simulink model "case7"  (R2024b)
settings: Solver=FixedStepAuto  StartTime=0  StopTime=1  FixedStep=1e-7  RelTol=1e-3
values from neighbouring files (symbols this model uses):
  SG_D_1_D = 0.01056    [IEEE9_case_parameters.m]    (also in case1_parameters.m; case2_parameters.m; case3_parameters.m; case4_parameters.m)
  SG_D_1_EnableSaturation = 0    [IEEE9_case_parameters.m]    (also in case1_parameters.m; case2_parameters.m; case3_parameters.m; case4_parameters.m)
  SG_D_1_f0 = 60    [IEEE9_case_parameters.m]    (also in case1_parameters.m; case2_parameters.m; case3_parameters.m; case4_parameters.m)
  SG_D_1_H = 7.5    [IEEE9_case_parameters.m]    (also in case1_parameters.m; case2_parameters.m; case3_parameters.m; case4_parameters.m)
  SG_D_1_K_A = 20    [IEEE9_case_parameters.m]    (also in case1_parameters.m; case2_parameters.m; case3_parameters.m; case4_parameters.m)
  SG_D_1_K_E = 1.000000e+1    (= 10)    [IEEE9_case_parameters.m]    (also in case1_parameters.m; case2_parameters.m; case3_parameters.m; case4_parameters.m)
  SG_D_1_K_F = 2.363    [IEEE9_case_parameters.m]    (also in case1_parameters.m; case2_parameters.m; case3_parameters.m; case4_parameters.m)
  SG_D_1_K_s = 0.5    [IEEE9_case_parameters.m]    (also in case1_parameters.m = 5; case2_parameters.m = 5; case3_parameters.m = 5; case4_parameters.m = 5)
  SG_D_1_R_a = 0.001088    [IEEE9_case_parameters.m]    (also in case1_parameters.m; case2_parameters.m; case3_parameters.m; case4_parameters.m)
  SG_D_1_S_A = 1    [IEEE9_case_parameters.m]    (also in case1_parameters.m; case2_parameters.m; case3_parameters.m; case4_parameters.m)
  SG_D_1_S_B = 0.103    [IEEE9_case_parameters.m]    (also in case1_parameters.m; case2_parameters.m; case3_parameters.m; case4_parameters.m)
  SG_D_1_S_N = 10.659857    [IEEE9_case_parameters.m]    (also in case1_parameters.m; case2_parameters.m; case3_parameters.m; case4_parameters.m)
  SG_D_1_SpeedPara = 200    [IEEE9_case_parameters.m]    (also in case1_parameters.m; case2_parameters.m; case3_parameters.m; case4_parameters.m)
  SG_D_1_T_0 = 0.720173    [IEEE9_case_parameters.m]    (also in case1_parameters.m = 0.755522; case2_parameters.m = 0.808931; case3_parameters.m = 0.869402; case4_parameters.m = 0.729316)
  SG_D_1_T_1 = 0.3    [IEEE9_case_parameters.m]    (also in case1_parameters.m; case2_parameters.m; case3_parameters.m; case4_parameters.m)
  SG_D_1_T_2 = 0.05    [IEEE9_case_parameters.m]    (also in case1_parameters.m; case2_parameters.m; case3_parameters.m; case4_parameters.m)
  SG_D_1_T_3 = 0.02    [IEEE9_case_parameters.m]    (also in case1_parameters.m; case2_parameters.m; case3_parameters.m; case4_parameters.m)
  SG_D_1_T_4 = 0.005    [IEEE9_case_parameters.m]    (also in case1_parameters.m; case2_parameters.m; case3_parameters.m; case4_parameters.m)
  SG_D_1_T_A = 0.02    [IEEE9_case_parameters.m]    (also in case1_parameters.m; case2_parameters.m; case3_parameters.m; case4_parameters.m)
  SG_D_1_T_dd = 8.000000e+0    (= 8)    [IEEE9_case_parameters.m]    (also in case1_parameters.m; case2_parameters.m; case3_parameters.m; case4_parameters.m)
  SG_D_1_T_ddd = 0.04    [IEEE9_case_parameters.m]    (also in case1_parameters.m; case2_parameters.m; case3_parameters.m; case4_parameters.m)
  SG_D_1_T_E = 0.314    [IEEE9_case_parameters.m]    (also in case1_parameters.m; case2_parameters.m; case3_parameters.m; case4_parameters.m)
  SG_D_1_T_F = 0.35    [IEEE9_case_parameters.m]    (also in case1_parameters.m; case2_parameters.m; case3_parameters.m; case4_parameters.m)
  SG_D_1_T_qd = 0.8    [IEEE9_case_parameters.m]    (also in case1_parameters.m; case2_parameters.m; case3_parameters.m; case4_parameters.m)
  SG_D_1_T_qdd = 0.02    [IEEE9_case_parameters.m]    (also in case1_parameters.m; case2_parameters.m; case3_parameters.m; case4_parameters.m)
  SG_D_1_T_speed = 0.1    [IEEE9_case_parameters.m]    (also in case1_parameters.m = 200; case2_parameters.m = 200; case3_parameters.m = 200; case4_parameters.m = 200)
  SG_D_1_T_w = 0.5    [IEEE9_case_parameters.m]    (also in case1_parameters.m; case2_parameters.m; case3_parameters.m; case4_parameters.m)
  SG_D_1_V_ref = 1.990276    [IEEE9_case_parameters.m]    (also in case1_parameters.m = 2.042296; case2_parameters.m = 2.051388; case3_parameters.m = 2.089584; case4_parameters.m = 2.01845)
  SG_D_1_w_ref = 376.991118    [IEEE9_case_parameters.m]    (also in case1_parameters.m; case2_parameters.m; case3_parameters.m; case4_parameters.m)
  SG_D_1_wb = 6.000000e+1    (= 60)    [IEEE9_case_parameters.m]    (also in case1_parameters.m; case2_parameters.m; case3_parameters.m; case4_parameters.m)
  SG_D_1_x_d = 1.9    [IEEE9_case_parameters.m]    (also in case1_parameters.m; case2_parameters.m; case3_parameters.m; case4_parameters.m)
  SG_D_1_x_dd = 0.302    [IEEE9_case_parameters.m]    (also in case1_parameters.m; case2_parameters.m; case3_parameters.m; case4_parameters.m)
  SG_D_1_x_ddd = 0.204    [IEEE9_case_parameters.m]    (also in case1_parameters.m; case2_parameters.m; case3_parameters.m; case4_parameters.m)
  SG_D_1_x_l = 0.05    [IEEE9_case_parameters.m]    (also in case1_parameters.m; case2_parameters.m; case3_parameters.m; case4_parameters.m)
  SG_D_1_x_q = 1.3    [IEEE9_case_parameters.m]    (also in case1_parameters.m; case2_parameters.m; case3_parameters.m; case4_parameters.m)
  SG_D_1_x_qd = 0.5    [IEEE9_case_parameters.m]    (also in case1_parameters.m; case2_parameters.m; case3_parameters.m; case4_parameters.m)
  SG_D_1_x_qdd = 0.3    [IEEE9_case_parameters.m]    (also in case1_parameters.m; case2_parameters.m; case3_parameters.m; case4_parameters.m)
  SG_D_2_D = 0.02    [IEEE9_case_parameters.m]    (also in case1_parameters.m; case2_parameters.m; case3_parameters.m; case4_parameters.m)
  SG_D_2_EnableSaturation = 0    [IEEE9_case_parameters.m]    (also in case1_parameters.m; case2_parameters.m; case3_parameters.m; case4_parameters.m)
  SG_D_2_f0 = 60    [IEEE9_case_parameters.m]    (also in case1_parameters.m; case2_parameters.m; case3_parameters.m; case4_parameters.m)
  SG_D_2_H = 8.000000e+0    (= 8)    [IEEE9_case_parameters.m]    (also in case1_parameters.m; case2_parameters.m; case3_parameters.m; case4_parameters.m)
  SG_D_2_K_A = 20    [IEEE9_case_parameters.m]    (also in case1_parameters.m; case2_parameters.m; case3_parameters.m; case4_parameters.m)
  SG_D_2_K_E = 1.000000e+1    (= 10)    [IEEE9_case_parameters.m]    (also in case1_parameters.m; case2_parameters.m; case3_parameters.m; case4_parameters.m)
  SG_D_2_K_F = 2.363    [IEEE9_case_parameters.m]    (also in case1_parameters.m; case2_parameters.m; case3_parameters.m; case4_parameters.m)
  SG_D_2_K_s = 0.5    [IEEE9_case_parameters.m]    (also in case1_parameters.m = 4; case2_parameters.m = 4; case3_parameters.m = 4; case4_parameters.m = 4)
  SG_D_2_R_a = 0.001088    [IEEE9_case_parameters.m]    (also in case1_parameters.m; case2_parameters.m; case3_parameters.m; case4_parameters.m)
  SG_D_2_S_A = 1    [IEEE9_case_parameters.m]    (also in case1_parameters.m; case2_parameters.m; case3_parameters.m; case4_parameters.m)
  SG_D_2_S_B = 0.103    [IEEE9_case_parameters.m]    (also in case1_parameters.m; case2_parameters.m; case3_parameters.m; case4_parameters.m)
  SG_D_2_S_N = 10.659857    [IEEE9_case_parameters.m]    (also in case1_parameters.m; case2_parameters.m; case3_parameters.m; case4_parameters.m)
  SG_D_2_SpeedPara = 200    [IEEE9_case_parameters.m]    (also in case1_parameters.m; case2_parameters.m; case3_parameters.m; case4_parameters.m)
  SG_D_2_T_0 = 1.632913    [IEEE9_case_parameters.m]    (also in case1_parameters.m = 1.632925; case2_parameters.m = 1.632915; case3_parameters.m = 1.632914; case4_parameters.m = 1.632927)
  SG_D_2_T_1 = 0.2    [IEEE9_case_parameters.m]    (also in case1_parameters.m; case2_parameters.m; case3_parameters.m; case4_parameters.m)
  SG_D_2_T_2 = 0.05    [IEEE9_case_parameters.m]    (also in case1_parameters.m; case2_parameters.m; case3_parameters.m; case4_parameters.m)
  SG_D_2_T_3 = 0.02    [IEEE9_case_parameters.m]    (also in case1_parameters.m; case2_parameters.m; case3_parameters.m; case4_parameters.m)
  SG_D_2_T_4 = 0.005    [IEEE9_case_parameters.m]    (also in case1_parameters.m; case2_parameters.m; case3_parameters.m; case4_parameters.m)
  SG_D_2_T_A = 0.02    [IEEE9_case_parameters.m]    (also in case1_parameters.m; case2_parameters.m; case3_parameters.m; case4_parameters.m)
  SG_D_2_T_dd = 7.9    [IEEE9_case_parameters.m]    (also in case1_parameters.m; case2_parameters.m; case3_parameters.m; case4_parameters.m)
  SG_D_2_T_ddd = 0.04    [IEEE9_case_parameters.m]    (also in case1_parameters.m; case2_parameters.m; case3_parameters.m; case4_parameters.m)
  SG_D_2_T_E = 0.314    [IEEE9_case_parameters.m]    (also in case1_parameters.m; case2_parameters.m; case3_parameters.m; case4_parameters.m)
  SG_D_2_T_F = 0.35    [IEEE9_case_parameters.m]    (also in case1_parameters.m; case2_parameters.m; case3_parameters.m; case4_parameters.m)
  SG_D_2_T_qd = 0.8    [IEEE9_case_parameters.m]    (also in case1_parameters.m; case2_parameters.m; case3_parameters.m; case4_parameters.m)
  SG_D_2_T_qdd = 0.015    [IEEE9_case_parameters.m]    (also in case1_parameters.m; case2_parameters.m; case3_parameters.m; case4_parameters.m)
  SG_D_2_T_speed = 0.1    [IEEE9_case_parameters.m]    (also in case1_parameters.m = 150; case2_parameters.m = 150; case3_parameters.m = 150; case4_parameters.m = 150)
  SG_D_2_T_w = 0.35    [IEEE9_case_parameters.m]    (also in case1_parameters.m; case2_parameters.m; case3_parameters.m; case4_parameters.m)
  SG_D_2_V_ref = 2.58547    [IEEE9_case_parameters.m]    (also in case1_parameters.m = 2.597896; case2_parameters.m = 2.587136; case3_parameters.m = 2.586042; case4_parameters.m = 2.599679)
  SG_D_2_w_ref = 376.991118    [IEEE9_case_parameters.m]    (also in case1_parameters.m; case2_parameters.m; case3_parameters.m; case4_parameters.m)
  SG_D_2_wb = 6.000000e+1    (= 60)    [IEEE9_case_parameters.m]    (also in case1_parameters.m; case2_parameters.m; case3_parameters.m; case4_parameters.m)
  SG_D_2_x_d = 1.8    [IEEE9_case_parameters.m]    (also in case1_parameters.m; case2_parameters.m; case3_parameters.m; case4_parameters.m)
  SG_D_2_x_dd = 0.302    [IEEE9_case_parameters.m]    (also in case1_parameters.m; case2_parameters.m; case3_parameters.m; case4_parameters.m)
  SG_D_2_x_ddd = 0.204    [IEEE9_case_parameters.m]    (also in case1_parameters.m; case2_parameters.m; case3_parameters.m; case4_parameters.m)
  SG_D_2_x_l = 0.05    [IEEE9_case_parameters.m]    (also in case1_parameters.m; case2_parameters.m; case3_parameters.m; case4_parameters.m)
  SG_D_2_x_q = 1.25    [IEEE9_case_parameters.m]    (also in case1_parameters.m; case2_parameters.m; case3_parameters.m; case4_parameters.m)
  SG_D_2_x_qd = 0.5    [IEEE9_case_parameters.m]    (also in case1_parameters.m; case2_parameters.m; case3_parameters.m; case4_parameters.m)
  SG_D_2_x_qdd = 0.3    [IEEE9_case_parameters.m]    (also in case1_parameters.m; case2_parameters.m; case3_parameters.m; case4_parameters.m)
  SG_D_3_D = 0.02    [IEEE9_case_parameters.m]    (also in case1_parameters.m; case2_parameters.m; case3_parameters.m; case4_parameters.m)
  SG_D_3_EnableSaturation = 0    [IEEE9_case_parameters.m]    (also in case1_parameters.m; case2_parameters.m; case3_parameters.m; case4_parameters.m)
  SG_D_3_f0 = 60    [IEEE9_case_parameters.m]    (also in case1_parameters.m; case2_parameters.m; case3_parameters.m; case4_parameters.m)
  SG_D_3_H = 7.7    [IEEE9_case_parameters.m]    (also in case1_parameters.m; case2_parameters.m; case3_parameters.m; case4_parameters.m)
  SG_D_3_K_A = 20    [IEEE9_case_parameters.m]    (also in case1_parameters.m; case2_parameters.m; case3_parameters.m; case4_parameters.m)
  SG_D_3_K_E = 1.000000e+1    (= 10)    [IEEE9_case_parameters.m]    (also in case1_parameters.m; case2_parameters.m; case3_parameters.m; case4_parameters.m)
  SG_D_3_K_F = 2.363    [IEEE9_case_parameters.m]    (also in case1_parameters.m; case2_parameters.m; case3_parameters.m; case4_parameters.m)
  SG_D_3_K_s = 0.2    [IEEE9_case_parameters.m]    (also in case1_parameters.m = 2; case2_parameters.m = 2; case3_parameters.m = 2; case4_parameters.m = 2)
  SG_D_3_R_a = 0.001088    [IEEE9_case_parameters.m]    (also in case1_parameters.m; case2_parameters.m; case3_parameters.m; case4_parameters.m)
  SG_D_3_S_A = 1    [IEEE9_case_parameters.m]    (also in case1_parameters.m; case2_parameters.m; case3_parameters.m; case4_parameters.m)
  SG_D_3_S_B = 0.103    [IEEE9_case_parameters.m]    (also in case1_parameters.m; case2_parameters.m; case3_parameters.m; case4_parameters.m)
  SG_D_3_S_N = 10.659857    [IEEE9_case_parameters.m]    (also in case1_parameters.m; case2_parameters.m; case3_parameters.m; case4_parameters.m)
  SG_D_3_SpeedPara = 200    [IEEE9_case_parameters.m]    (also in case1_parameters.m; case2_parameters.m; case3_parameters.m; case4_parameters.m)
  SG_D_3_T_0 = 0.850788    [IEEE9_case_parameters.m]    (also in case1_parameters.m = 0.850786; case2_parameters.m = 0.850787; case3_parameters.m; case4_parameters.m = 0.850786)
  SG_D_3_T_1 = 0.2    [IEEE9_case_parameters.m]    (also in case1_parameters.m; case2_parameters.m; case3_parameters.m; case4_parameters.m)
  SG_D_3_T_2 = 0.05    [IEEE9_case_parameters.m]    (also in case1_parameters.m; case2_parameters.m; case3_parameters.m; case4_parameters.m)
  SG_D_3_T_3 = 0.02    [IEEE9_case_parameters.m]    (also in case1_parameters.m; case2_parameters.m; case3_parameters.m; case4_parameters.m)
  SG_D_3_T_4 = 0.005    [IEEE9_case_parameters.m]    (also in case1_parameters.m; case2_parameters.m; case3_parameters.m; case4_parameters.m)
  SG_D_3_T_A = 0.02    [IEEE9_case_parameters.m]    (also in case1_parameters.m; case2_parameters.m; case3_parameters.m; case4_parameters.m)
  SG_D_3_T_dd = 8.1    [IEEE9_case_parameters.m]    (also in case1_parameters.m; case2_parameters.m; case3_parameters.m; case4_parameters.m)
  SG_D_3_T_ddd = 0.04    [IEEE9_case_parameters.m]    (also in case1_parameters.m; case2_parameters.m; case3_parameters.m; case4_parameters.m)
  SG_D_3_T_E = 0.314    [IEEE9_case_parameters.m]    (also in case1_parameters.m; case2_parameters.m; case3_parameters.m; case4_parameters.m)
  SG_D_3_T_F = 0.35    [IEEE9_case_parameters.m]    (also in case1_parameters.m; case2_parameters.m; case3_parameters.m; case4_parameters.m)
  SG_D_3_T_qd = 0.8    [IEEE9_case_parameters.m]    (also in case1_parameters.m; case2_parameters.m; case3_parameters.m; case4_parameters.m)
  SG_D_3_T_qdd = 0.015    [IEEE9_case_parameters.m]    (also in case1_parameters.m; case2_parameters.m; case3_parameters.m; case4_parameters.m)
  SG_D_3_T_speed = 0.1    [IEEE9_case_parameters.m]    (also in case1_parameters.m = 180; case2_parameters.m = 180; case3_parameters.m = 180; case4_parameters.m = 180)
  SG_D_3_T_w = 0.4    [IEEE9_case_parameters.m]    (also in case1_parameters.m; case2_parameters.m; case3_parameters.m; case4_parameters.m)
  SG_D_3_V_ref = 1.892727    [IEEE9_case_parameters.m]    (also in case1_parameters.m = 1.906439; case2_parameters.m = 1.895535; case3_parameters.m = 1.892105; case4_parameters.m = 1.906598)
  SG_D_3_w_ref = 376.991118    [IEEE9_case_parameters.m]    (also in case1_parameters.m; case2_parameters.m; case3_parameters.m; case4_parameters.m)
  SG_D_3_wb = 6.000000e+1    (= 60)    [IEEE9_case_parameters.m]    (also in case1_parameters.m; case2_parameters.m; case3_parameters.m; case4_parameters.m)
  SG_D_3_x_d = 1.85    [IEEE9_case_parameters.m]    (also in case1_parameters.m; case2_parameters.m; case3_parameters.m; case4_parameters.m)
  SG_D_3_x_dd = 0.302    [IEEE9_case_parameters.m]    (also in case1_parameters.m; case2_parameters.m; case3_parameters.m; case4_parameters.m)
  SG_D_3_x_ddd = 0.204    [IEEE9_case_parameters.m]    (also in case1_parameters.m; case2_parameters.m; case3_parameters.m; case4_parameters.m)
  SG_D_3_x_l = 0.05    [IEEE9_case_parameters.m]    (also in case1_parameters.m; case2_parameters.m; case3_parameters.m; case4_parameters.m)
  SG_D_3_x_q = 1.2    [IEEE9_case_parameters.m]    (also in case1_parameters.m; case2_parameters.m; case3_parameters.m; case4_parameters.m)
  SG_D_3_x_qd = 0.5    [IEEE9_case_parameters.m]    (also in case1_parameters.m; case2_parameters.m; case3_parameters.m; case4_parameters.m)
  SG_D_3_x_qdd = 0.3    [IEEE9_case_parameters.m]    (also in case1_parameters.m; case2_parameters.m; case3_parameters.m; case4_parameters.m)
(part 2 of 12)

== system case7/SG_D_2 ==
  v_d_SG_D_2 : Inport
  v_q_SG_D_2 : Inport  Port=2
  E_fd_SG_D_2 : Integrator  InitialCondition=3.144075614664211
  Px_1_SG_D_2 : Integrator  InitialCondition=0.0
  Px_2_SG_D_2 : Integrator  InitialCondition=0.0
  Px_3_SG_D_2 : Integrator  InitialCondition=-3.1909481078527976e-25
  R_f_SG_D_2 : Integrator  InitialCondition=21.227001935575803
  T_e_SG_D_2_block : Subsystem
  T_m_SG_D_2 : Integrator  InitialCondition=1.632903124801411
  V_f_SG_D_2 : Integrator  InitialCondition=31.44075614664211
  d_E_fd_SG_D_2_block : Subsystem
  d_Px_1_SG_D_2_block : Subsystem
  d_Px_2_SG_D_2_block : Subsystem
  d_Px_3_SG_D_2_block : Subsystem
  d_R_f_SG_D_2_block : Subsystem
  d_T_m_SG_D_2_block : Subsystem
  d_V_f_SG_D_2_block : Subsystem
  d_psi_1d_SG_D_2_block : Subsystem
  d_psi_d_SG_D_2_block : Subsystem
  d_psi_fd_SG_D_2_block : Subsystem
  d_psi_gq_SG_D_2_block : Subsystem
  d_psi_kq_SG_D_2_block : Subsystem
  d_psi_q_SG_D_2_block : Subsystem
  d_theta_SG_D_2_block : Subsystem
  d_w_SG_D_2_block : Subsystem
  i_d_SG_D_2_block : Subsystem
  i_q_SG_D_2_block : Subsystem
  psi_1d_SG_D_2 : Integrator  InitialCondition=0.561322457114984
  psi_d_SG_D_2 : Integrator  InitialCondition=0.48752950975643444
  psi_fd_SG_D_2 : Integrator  InitialCondition=0.9332389118020725
  psi_gq_SG_D_2 : Integrator  InitialCondition=0.5250822846595283
  psi_kq_SG_D_2 : Integrator  InitialCondition=-0.8401316554552454
  psi_q_SG_D_2 : Integrator  InitialCondition=-0.8751371410992139
  theta_SG_D_2 : Integrator  InitialCondition=1.2331134465315912
  theta_SG_D_2_out_block : Subsystem
  w_SG_D_2 : Integrator  InitialCondition=376.99111843077515
  w_SG_D_2_out_block : Subsystem
  i_d_SG_D_2 : Outport
  i_q_SG_D_2 : Outport  Port=2
  T_e_SG_D_2 : Outport  Port=3
  w_SG_D_2_out : Outport  Port=4
  theta_SG_D_2_out : Outport  Port=5
  wires:
  T_e_SG_D_2_block/1(Blockout_T_e_SG_D_2_730cc) -> T_e_SG_D_2/1
  d_Px_2_SG_D_2_block/1(Blockout_d_Px_2_SG_D_2_f4188) -> Px_2_SG_D_2/1
  d_T_m_SG_D_2_block/1(Blockout_d_T_m_SG_D_2_7fa4d) -> T_m_SG_D_2/1
  w_SG_D_2/1 -> d_psi_d_SG_D_2_block/9(State_w_SG_D_2_79fa8), d_psi_q_SG_D_2_block/9(State_w_SG_D_2_933ea), d_w_SG_D_2_block/1(State_w_SG_D_2_9254d), d_V_f_SG_D_2_block/8(State_w_SG_D_2_be721), d_V_f_SG_D_2_block/13(State_w_SG_D_2_eddc0), d_Px_3_SG_D_2_block/6(State_w_SG_D_2_022fa), d_Px_2_SG_D_2_block/4(State_w_SG_D_2_465a1), w_SG_D_2_out_block/1(State_w_SG_D_2_7ae1a), d_Px_1_SG_D_2_block/2(State_w_SG_D_2_7a34c), d_T_m_SG_D_2_block/1(State_w_SG_D_2_7be82), d_theta_SG_D_2_block/1(State_w_SG_D_2_14bd2)
  d_Px_3_SG_D_2_block/1(Blockout_d_Px_3_SG_D_2_173a6) -> Px_3_SG_D_2/1
  psi_kq_SG_D_2/1 -> d_psi_q_SG_D_2_block/2(State_psi_kq_SG_D_2_21fa1), d_psi_gq_SG_D_2_block/3(State_psi_kq_SG_D_2_14835), d_psi_gq_SG_D_2_block/5(State_psi_kq_SG_D_2_a8c2a), d_psi_kq_SG_D_2_block/4(State_psi_kq_SG_D_2_d9628), d_w_SG_D_2_block/5(State_psi_kq_SG_D_2_98079), d_V_f_SG_D_2_block/10(State_psi_kq_SG_D_2_6eadf), i_d_SG_D_2_block/2(State_psi_kq_SG_D_2_f7ad5), d_psi_gq_SG_D_2_block/8(State_psi_kq_SG_D_2_1a38a), i_q_SG_D_2_block/2(State_psi_kq_SG_D_2_111a7), d_psi_kq_SG_D_2_block/2(State_psi_kq_SG_D_2_1ae2e), T_e_SG_D_2_block/3(State_psi_kq_SG_D_2_7391f)
  d_Px_1_SG_D_2_block/1(Blockout_d_Px_1_SG_D_2_2c2a9) -> Px_1_SG_D_2/1
  d_theta_SG_D_2_block/1(Blockout_d_theta_SG_D_2_87c37) -> theta_SG_D_2/1
  psi_q_SG_D_2/1 -> d_psi_d_SG_D_2_block/8(State_psi_q_SG_D_2_5b767), d_psi_q_SG_D_2_block/3(State_psi_q_SG_D_2_91656), d_psi_gq_SG_D_2_block/9(State_psi_q_SG_D_2_46358), d_psi_kq_SG_D_2_block/5(State_psi_q_SG_D_2_5421a), d_w_SG_D_2_block/7(State_psi_q_SG_D_2_98409), d_w_SG_D_2_block/6(State_psi_q_SG_D_2_b528a), i_d_SG_D_2_block/3(State_psi_q_SG_D_2_5a7c7), d_psi_gq_SG_D_2_block/6(State_psi_q_SG_D_2_e2d01), d_V_f_SG_D_2_block/7(State_psi_q_SG_D_2_852ab), i_q_SG_D_2_block/3(State_psi_q_SG_D_2_3ac1e), d_V_f_SG_D_2_block/11(State_psi_q_SG_D_2_e8b59), T_e_SG_D_2_block/5(State_psi_q_SG_D_2_7a09c), T_e_SG_D_2_block/4(State_psi_q_SG_D_2_f6431)
  w_SG_D_2_out_block/1(Blockout_w_SG_D_2_out_61ea1) -> w_SG_D_2_out/1
  psi_fd_SG_D_2/1 -> d_psi_fd_SG_D_2_block/2(State_psi_fd_SG_D_2_c8c63), d_psi_fd_SG_D_2_block/4(State_psi_fd_SG_D_2_c9eab), d_psi_fd_SG_D_2_block/7(State_psi_fd_SG_D_2_d23df), d_psi_fd_SG_D_2_block/10(State_psi_fd_SG_D_2_17d9a), d_psi_1d_SG_D_2_block/2(State_psi_fd_SG_D_2_7f283), d_V_f_SG_D_2_block/6(State_psi_fd_SG_D_2_4efc9), i_d_SG_D_2_block/7(State_psi_fd_SG_D_2_e8aea), d_w_SG_D_2_block/10(State_psi_fd_SG_D_2_5b538), d_psi_d_SG_D_2_block/3(State_psi_fd_SG_D_2_079ef), d_psi_1d_SG_D_2_block/5(State_psi_fd_SG_D_2_c6554), i_q_SG_D_2_block/7(State_psi_fd_SG_D_2_e2311), T_e_SG_D_2_block/8(State_psi_fd_SG_D_2_f8f9e)
  psi_gq_SG_D_2/1 -> d_psi_q_SG_D_2_block/1(State_psi_gq_SG_D_2_7156c), d_psi_gq_SG_D_2_block/1(State_psi_gq_SG_D_2_04112), d_psi_gq_SG_D_2_block/2(State_psi_gq_SG_D_2_2f535), d_psi_gq_SG_D_2_block/4(State_psi_gq_SG_D_2_fc0a1), d_psi_kq_SG_D_2_block/1(State_psi_gq_SG_D_2_30603), d_psi_kq_SG_D_2_block/3(State_psi_gq_SG_D_2_ebfa7), d_w_SG_D_2_block/4(State_psi_gq_SG_D_2_dac01), d_V_f_SG_D_2_block/9(State_psi_gq_SG_D_2_b910f), i_q_SG_D_2_block/1(State_psi_gq_SG_D_2_9874f), d_psi_gq_SG_D_2_block/7(State_psi_gq_SG_D_2_2f96e), T_e_SG_D_2_block/2(State_psi_gq_SG_D_2_7da5e), i_d_SG_D_2_block/1(State_psi_gq_SG_D_2_2ca68)
  T_m_SG_D_2/1 -> d_T_m_SG_D_2_block/2(State_T_m_SG_D_2_01c83), d_w_SG_D_2_block/2(State_T_m_SG_D_2_4b7e4)
  v_d_SG_D_2/1 -> d_psi_d_SG_D_2_block/4(Input_v_d_SG_D_2_793e9), d_psi_q_SG_D_2_block/4(Input_v_d_SG_D_2_12f1d)
  psi_1d_SG_D_2/1 -> d_psi_fd_SG_D_2_block/3(State_psi_1d_SG_D_2_57e67), d_psi_fd_SG_D_2_block/5(State_psi_1d_SG_D_2_8d090), d_psi_d_SG_D_2_block/1(State_psi_1d_SG_D_2_39a46), d_psi_1d_SG_D_2_block/3(State_psi_1d_SG_D_2_a8fff), d_w_SG_D_2_block/8(State_psi_1d_SG_D_2_79084), d_V_f_SG_D_2_block/4(State_psi_1d_SG_D_2_fddcb), d_psi_1d_SG_D_2_block/1(State_psi_1d_SG_D_2_3a9a3), i_d_SG_D_2_block/5(State_psi_1d_SG_D_2_3541a), d_psi_fd_SG_D_2_block/8(State_psi_1d_SG_D_2_76ec9), T_e_SG_D_2_block/6(State_psi_1d_SG_D_2_55ddd), i_q_SG_D_2_block/5(State_psi_1d_SG_D_2_f6d17)
  d_V_f_SG_D_2_block/1(Blockout_d_V_f_SG_D_2_0f1c6) -> V_f_SG_D_2/1
  v_q_SG_D_2/1 -> d_psi_d_SG_D_2_block/6(Input_v_q_SG_D_2_3f1f5), d_psi_q_SG_D_2_block/6(Input_v_q_SG_D_2_7d1d1)
  theta_SG_D_2/1 -> d_psi_d_SG_D_2_block/5(State_theta_SG_D_2_659a4), d_psi_d_SG_D_2_block/7(State_theta_SG_D_2_bf2b8), d_psi_q_SG_D_2_block/5(State_theta_SG_D_2_c47ee), i_d_SG_D_2_block/4(State_theta_SG_D_2_df193), i_q_SG_D_2_block/8(State_theta_SG_D_2_15c5e), i_d_SG_D_2_block/8(State_theta_SG_D_2_1457d), theta_SG_D_2_out_block/1(State_theta_SG_D_2_7f9e2), d_psi_q_SG_D_2_block/7(State_theta_SG_D_2_7c757), i_q_SG_D_2_block/4(State_theta_SG_D_2_a60df)
  Px_2_SG_D_2/1 -> d_Px_3_SG_D_2_block/2(State_Px_2_SG_D_2_71991), d_Px_2_SG_D_2_block/1(State_Px_2_SG_D_2_9a1df), d_Px_3_SG_D_2_block/3(State_Px_2_SG_D_2_f02e6)
  Px_1_SG_D_2/1 -> d_Px_1_SG_D_2_block/1(State_Px_1_SG_D_2_f4101), d_Px_2_SG_D_2_block/2(State_Px_1_SG_D_2_e97bf), d_Px_2_SG_D_2_block/3(State_Px_1_SG_D_2_8c4e1), d_Px_3_SG_D_2_block/4(State_Px_1_SG_D_2_7e74e), d_Px_3_SG_D_2_block/5(State_Px_1_SG_D_2_1642d)
  i_d_SG_D_2_block/1(Blockout_i_d_SG_D_2_adf62) -> i_d_SG_D_2/1
  psi_d_SG_D_2/1 -> d_psi_fd_SG_D_2_block/6(State_psi_d_SG_D_2_c1fee), d_psi_fd_SG_D_2_block/9(State_psi_d_SG_D_2_fe578), d_psi_d_SG_D_2_block/2(State_psi_d_SG_D_2_1ecaf), d_psi_q_SG_D_2_block/8(State_psi_d_SG_D_2_b6b26), d_psi_1d_SG_D_2_block/4(State_psi_d_SG_D_2_2213a), d_w_SG_D_2_block/9(State_psi_d_SG_D_2_b6680), d_w_SG_D_2_block/3(State_psi_d_SG_D_2_c41d8), d_V_f_SG_D_2_block/5(State_psi_d_SG_D_2_5d6e4), d_V_f_SG_D_2_block/12(State_psi_d_SG_D_2_e6df7), i_q_SG_D_2_block/6(State_psi_d_SG_D_2_87493), i_d_SG_D_2_block/6(State_psi_d_SG_D_2_d4d6e), T_e_SG_D_2_block/7(State_psi_d_SG_D_2_ae3de), T_e_SG_D_2_block/1(State_psi_d_SG_D_2_bf269)
  d_psi_kq_SG_D_2_block/1(Blockout_d_psi_kq_SG_D_2_9fcf6) -> psi_kq_SG_D_2/1
  d_R_f_SG_D_2_block/1(Blockout_d_R_f_SG_D_2_b27f4) -> R_f_SG_D_2/1
  d_psi_gq_SG_D_2_block/1(Blockout_d_psi_gq_SG_D_2_e8d92) -> psi_gq_SG_D_2/1
  i_q_SG_D_2_block/1(Blockout_i_q_SG_D_2_2255f) -> i_q_SG_D_2/1
  d_w_SG_D_2_block/1(Blockout_d_w_SG_D_2_dce26) -> w_SG_D_2/1
  d_psi_d_SG_D_2_block/1(Blockout_d_psi_d_SG_D_2_9d3b5) -> psi_d_SG_D_2/1
  d_psi_q_SG_D_2_block/1(Blockout_d_psi_q_SG_D_2_62d90) -> psi_q_SG_D_2/1
  d_psi_1d_SG_D_2_block/1(Blockout_d_psi_1d_SG_D_2_9a5fd) -> psi_1d_SG_D_2/1
  R_f_SG_D_2/1 -> d_V_f_SG_D_2_block/2(State_R_f_SG_D_2_2bc07), d_R_f_SG_D_2_block/2(State_R_f_SG_D_2_2054a)
  theta_SG_D_2_out_block/1(Blockout_theta_SG_D_2_out_31e40) -> theta_SG_D_2_out/1
  V_f_SG_D_2/1 -> d_V_f_SG_D_2_block/14(State_V_f_SG_D_2_b87cd), d_E_fd_SG_D_2_block/2(State_V_f_SG_D_2_83e9f)
  Px_3_SG_D_2/1 -> d_V_f_SG_D_2_block/3(State_Px_3_SG_D_2_b3414), d_Px_3_SG_D_2_block/1(State_Px_3_SG_D_2_9d0f6)
  d_E_fd_SG_D_2_block/1(Blockout_d_E_fd_SG_D_2_7fc5f) -> E_fd_SG_D_2/1
  E_fd_SG_D_2/1 -> d_V_f_SG_D_2_block/1(State_E_fd_SG_D_2_fa01a), d_E_fd_SG_D_2_block/1(State_E_fd_SG_D_2_ac2d4), d_psi_fd_SG_D_2_block/1(State_E_fd_SG_D_2_6abd7), d_R_f_SG_D_2_block/1(State_E_fd_SG_D_2_7a8b0)
  d_psi_fd_SG_D_2_block/1(Blockout_d_psi_fd_SG_D_2_d186f) -> psi_fd_SG_D_2/1

== system case7/SG_D_3 ==
  v_d_SG_D_3 : Inport
  v_q_SG_D_3 : Inport  Port=2
  E_fd_SG_D_3 : Integrator  InitialCondition=1.752988789914741
  Px_1_SG_D_3 : Integrator  InitialCondition=0.0
  Px_2_SG_D_3 : Integrator  InitialCondition=0.0
  Px_3_SG_D_3 : Integrator  InitialCondition=-1.823793620772198e-24
  R_f_SG_D_3 : Integrator  InitialCondition=11.835178601624381
  T_e_SG_D_3_block : Subsystem
  T_m_SG_D_3 : Integrator  InitialCondition=0.8507912713205479
  V_f_SG_D_3 : Integrator  InitialCondition=17.52988789914741
  d_E_fd_SG_D_3_block : Subsystem
  d_Px_1_SG_D_3_block : Subsystem
  d_Px_2_SG_D_3_block : Subsystem
  d_Px_3_SG_D_3_block : Subsystem
  d_R_f_SG_D_3_block : Subsystem
  d_T_m_SG_D_3_block : Subsystem
  d_V_f_SG_D_3_block : Subsystem
  d_psi_1d_SG_D_3_block : Subsystem
  d_psi_d_SG_D_3_block : Subsystem
  d_psi_fd_SG_D_3_block : Subsystem
  d_psi_gq_SG_D_3_block : Subsystem
  d_psi_kq_SG_D_3_block : Subsystem
  d_psi_q_SG_D_3_block : Subsystem
  d_theta_SG_D_3_block : Subsystem
  d_w_SG_D_3_block : Subsystem
  i_d_SG_D_3_block : Subsystem
  i_q_SG_D_3_block : Subsystem
  psi_1d_SG_D_3 : Integrator  InitialCondition=0.6989053679197881
  psi_d_SG_D_3 : Integrator  InitialCondition=0.6696252728643726
  psi_fd_SG_D_3 : Integrator  InitialCondition=0.8464770469990816
  psi_gq_SG_D_3 : Integrator  InitialCondition=0.4339672469609975
  psi_kq_SG_D_3 : Integrator  InitialCondition=-0.7129461914359245
  psi_q_SG_D_3 : Integrator  InitialCondition=-0.7439438519331386
  theta_SG_D_3 : Integrator  InitialCondition=0.9232913969642249
  theta_SG_D_3_out_block : Subsystem
  w_SG_D_3 : Integrator  InitialCondition=376.99111843077515
  w_SG_D_3_out_block : Subsystem
  i_d_SG_D_3 : Outport
  i_q_SG_D_3 : Outport  Port=2
  T_e_SG_D_3 : Outport  Port=3
  w_SG_D_3_out : Outport  Port=4
  theta_SG_D_3_out : Outport  Port=5
  wires:
  d_Px_1_SG_D_3_block/1(Blockout_d_Px_1_SG_D_3_f80fa) -> Px_1_SG_D_3/1
  w_SG_D_3/1 -> d_psi_d_SG_D_3_block/9(State_w_SG_D_3_0f458), d_psi_q_SG_D_3_block/9(State_w_SG_D_3_e996e), d_w_SG_D_3_block/1(State_w_SG_D_3_49d00), d_V_f_SG_D_3_block/13(State_w_SG_D_3_9a9fd), d_V_f_SG_D_3_block/8(State_w_SG_D_3_07b93), d_T_m_SG_D_3_block/1(State_w_SG_D_3_b61f5), d_theta_SG_D_3_block/1(State_w_SG_D_3_e06ca), d_Px_1_SG_D_3_block/2(State_w_SG_D_3_68398), d_Px_2_SG_D_3_block/4(State_w_SG_D_3_fe34a), w_SG_D_3_out_block/1(State_w_SG_D_3_59408), d_Px_3_SG_D_3_block/6(State_w_SG_D_3_03f21)
  d_T_m_SG_D_3_block/1(Blockout_d_T_m_SG_D_3_419d3) -> T_m_SG_D_3/1
  d_w_SG_D_3_block/1(Blockout_d_w_SG_D_3_e861c) -> w_SG_D_3/1
  Px_1_SG_D_3/1 -> d_Px_1_SG_D_3_block/1(State_Px_1_SG_D_3_f55d0), d_Px_2_SG_D_3_block/2(State_Px_1_SG_D_3_910c8), d_Px_3_SG_D_3_block/4(State_Px_1_SG_D_3_9cfb8), d_Px_2_SG_D_3_block/3(State_Px_1_SG_D_3_d78a2), d_Px_3_SG_D_3_block/5(State_Px_1_SG_D_3_6302b)
  d_theta_SG_D_3_block/1(Blockout_d_theta_SG_D_3_abfc2) -> theta_SG_D_3/1
  d_Px_2_SG_D_3_block/1(Blockout_d_Px_2_SG_D_3_8d5d5) -> Px_2_SG_D_3/1
  R_f_SG_D_3/1 -> d_V_f_SG_D_3_block/2(State_R_f_SG_D_3_7b882), d_R_f_SG_D_3_block/2(State_R_f_SG_D_3_2f1ad)
  w_SG_D_3_out_block/1(Blockout_w_SG_D_3_out_9dbeb) -> w_SG_D_3_out/1
  d_Px_3_SG_D_3_block/1(Blockout_d_Px_3_SG_D_3_7ae60) -> Px_3_SG_D_3/1
  d_psi_kq_SG_D_3_block/1(Blockout_d_psi_kq_SG_D_3_d1c2e) -> psi_kq_SG_D_3/1
  psi_1d_SG_D_3/1 -> d_psi_fd_SG_D_3_block/3(State_psi_1d_SG_D_3_05d9c), d_psi_fd_SG_D_3_block/8(State_psi_1d_SG_D_3_2ff45), d_psi_fd_SG_D_3_block/5(State_psi_1d_SG_D_3_135f0), d_psi_d_SG_D_3_block/1(State_psi_1d_SG_D_3_ab585), d_psi_1d_SG_D_3_block/3(State_psi_1d_SG_D_3_8936f), d_w_SG_D_3_block/8(State_psi_1d_SG_D_3_b8ac8), d_psi_1d_SG_D_3_block/1(State_psi_1d_SG_D_3_0b4b8), i_d_SG_D_3_block/5(State_psi_1d_SG_D_3_0e0c9), i_q_SG_D_3_block/5(State_psi_1d_SG_D_3_b9ac9), T_e_SG_D_3_block/6(State_psi_1d_SG_D_3_4e6ed), d_V_f_SG_D_3_block/4(State_psi_1d_SG_D_3_9321f)
  v_d_SG_D_3/1 -> d_psi_d_SG_D_3_block/4(Input_v_d_SG_D_3_0a2ba), d_psi_q_SG_D_3_block/4(Input_v_d_SG_D_3_f4c2d)
  v_q_SG_D_3/1 -> d_psi_d_SG_D_3_block/6(Input_v_q_SG_D_3_ba6ff), d_psi_q_SG_D_3_block/6(Input_v_q_SG_D_3_303a8)
  psi_q_SG_D_3/1 -> d_psi_d_SG_D_3_block/8(State_psi_q_SG_D_3_1f0c4), d_psi_q_SG_D_3_block/3(State_psi_q_SG_D_3_7fdb8), d_psi_gq_SG_D_3_block/6(State_psi_q_SG_D_3_4f3e1), d_psi_kq_SG_D_3_block/5(State_psi_q_SG_D_3_3b0fa), d_w_SG_D_3_block/6(State_psi_q_SG_D_3_9d6c4), d_w_SG_D_3_block/7(State_psi_q_SG_D_3_0cb4b), d_V_f_SG_D_3_block/11(State_psi_q_SG_D_3_fc547), d_psi_gq_SG_D_3_block/9(State_psi_q_SG_D_3_b59db), i_d_SG_D_3_block/3(State_psi_q_SG_D_3_af60f), i_q_SG_D_3_block/3(State_psi_q_SG_D_3_80977), d_V_f_SG_D_3_block/7(State_psi_q_SG_D_3_16277), T_e_SG_D_3_block/4(State_psi_q_SG_D_3_08b99), T_e_SG_D_3_block/5(State_psi_q_SG_D_3_6cef3)
  T_m_SG_D_3/1 -> d_T_m_SG_D_3_block/2(State_T_m_SG_D_3_9a3dd), d_w_SG_D_3_block/2(State_T_m_SG_D_3_f04ec)
  theta_SG_D_3/1 -> d_psi_d_SG_D_3_block/5(State_theta_SG_D_3_52860), d_psi_d_SG_D_3_block/7(State_theta_SG_D_3_fae54), i_d_SG_D_3_block/8(State_theta_SG_D_3_4b034), i_d_SG_D_3_block/4(State_theta_SG_D_3_14959), i_q_SG_D_3_block/4(State_theta_SG_D_3_7a7eb), d_psi_q_SG_D_3_block/7(State_theta_SG_D_3_98ce1), i_q_SG_D_3_block/8(State_theta_SG_D_3_559de), theta_SG_D_3_out_block/1(State_theta_SG_D_3_a405f), d_psi_q_SG_D_3_block/5(State_theta_SG_D_3_e0e57)
  psi_d_SG_D_3/1 -> d_psi_fd_SG_D_3_block/6(State_psi_d_SG_D_3_e7d35), d_psi_fd_SG_D_3_block/9(State_psi_d_SG_D_3_5ac00), d_psi_d_SG_D_3_block/2(State_psi_d_SG_D_3_41343), d_psi_q_SG_D_3_block/8(State_psi_d_SG_D_3_074a8), d_psi_1d_SG_D_3_block/4(State_psi_d_SG_D_3_ea1f7), d_V_f_SG_D_3_block/5(State_psi_d_SG_D_3_27134), d_w_SG_D_3_block/9(State_psi_d_SG_D_3_21482), d_V_f_SG_D_3_block/12(State_psi_d_SG_D_3_2d4a5), d_w_SG_D_3_block/3(State_psi_d_SG_D_3_b4422), i_q_SG_D_3_block/6(State_psi_d_SG_D_3_372cf), i_d_SG_D_3_block/6(State_psi_d_SG_D_3_94a65), T_e_SG_D_3_block/1(State_psi_d_SG_D_3_21043), T_e_SG_D_3_block/7(State_psi_d_SG_D_3_2ba64)
  Px_2_SG_D_3/1 -> d_Px_2_SG_D_3_block/1(State_Px_2_SG_D_3_db3bd), d_Px_3_SG_D_3_block/2(State_Px_2_SG_D_3_e7342), d_Px_3_SG_D_3_block/3(State_Px_2_SG_D_3_4c474)
  psi_fd_SG_D_3/1 -> d_psi_fd_SG_D_3_block/2(State_psi_fd_SG_D_3_d8879), d_psi_fd_SG_D_3_block/4(State_psi_fd_SG_D_3_36249), d_psi_fd_SG_D_3_block/7(State_psi_fd_SG_D_3_10381), d_psi_fd_SG_D_3_block/10(State_psi_fd_SG_D_3_ba8dd), d_psi_d_SG_D_3_block/3(State_psi_fd_SG_D_3_7e2f5), d_psi_1d_SG_D_3_block/5(State_psi_fd_SG_D_3_e1882), d_w_SG_D_3_block/10(State_psi_fd_SG_D_3_a31e3), d_psi_1d_SG_D_3_block/2(State_psi_fd_SG_D_3_02f28), i_d_SG_D_3_block/7(State_psi_fd_SG_D_3_81ff2), d_V_f_SG_D_3_block/6(State_psi_fd_SG_D_3_2f745), i_q_SG_D_3_block/7(State_psi_fd_SG_D_3_73d0e), T_e_SG_D_3_block/8(State_psi_fd_SG_D_3_03760)
  psi_kq_SG_D_3/1 -> d_psi_q_SG_D_3_block/2(State_psi_kq_SG_D_3_940c9), d_psi_gq_SG_D_3_block/3(State_psi_kq_SG_D_3_33b37), d_w_SG_D_3_block/5(State_psi_kq_SG_D_3_26e8a), d_psi_gq_SG_D_3_block/5(State_psi_kq_SG_D_3_ef6ad), d_psi_gq_SG_D_3_block/8(State_psi_kq_SG_D_3_15928), d_psi_kq_SG_D_3_block/4(State_psi_kq_SG_D_3_904ed), i_d_SG_D_3_block/2(State_psi_kq_SG_D_3_f6ce0), d_V_f_SG_D_3_block/10(State_psi_kq_SG_D_3_71eef), d_psi_kq_SG_D_3_block/2(State_psi_kq_SG_D_3_60998), i_q_SG_D_3_block/2(State_psi_kq_SG_D_3_8c674), T_e_SG_D_3_block/3(State_psi_kq_SG_D_3_78f61)
  psi_gq_SG_D_3/1 -> d_psi_q_SG_D_3_block/1(State_psi_gq_SG_D_3_f880b), d_psi_gq_SG_D_3_block/2(State_psi_gq_SG_D_3_4ee3d), d_psi_gq_SG_D_3_block/4(State_psi_gq_SG_D_3_62341), d_psi_kq_SG_D_3_block/1(State_psi_gq_SG_D_3_cecd3), d_psi_kq_SG_D_3_block/3(State_psi_gq_SG_D_3_2a36c), d_psi_gq_SG_D_3_block/7(State_psi_gq_SG_D_3_01274), d_w_SG_D_3_block/4(State_psi_gq_SG_D_3_3cfd1), d_psi_gq_SG_D_3_block/1(State_psi_gq_SG_D_3_42a13), i_d_SG_D_3_block/1(State_psi_gq_SG_D_3_6922b), i_q_SG_D_3_block/1(State_psi_gq_SG_D_3_a9771), T_e_SG_D_3_block/2(State_psi_gq_SG_D_3_33d2c), d_V_f_SG_D_3_block/9(State_psi_gq_SG_D_3_4d40d)
  d_psi_q_SG_D_3_block/1(Blockout_d_psi_q_SG_D_3_20592) -> psi_q_SG_D_3/1
  d_R_f_SG_D_3_block/1(Blockout_d_R_f_SG_D_3_e162d) -> R_f_SG_D_3/1
  theta_SG_D_3_out_block/1(Blockout_theta_SG_D_3_out_42e30) -> theta_SG_D_3_out/1
  d_V_f_SG_D_3_block/1(Blockout_d_V_f_SG_D_3_6b0a5) -> V_f_SG_D_3/1
  i_d_SG_D_3_block/1(Blockout_i_d_SG_D_3_97111) -> i_d_SG_D_3/1
  d_psi_d_SG_D_3_block/1(Blockout_d_psi_d_SG_D_3_1dab3) -> psi_d_SG_D_3/1
  d_psi_1d_SG_D_3_block/1(Blockout_d_psi_1d_SG_D_3_24fb6) -> psi_1d_SG_D_3/1
  i_q_SG_D_3_block/1(Blockout_i_q_SG_D_3_34aae) -> i_q_SG_D_3/1
  T_e_SG_D_3_block/1(Blockout_T_e_SG_D_3_4c18a) -> T_e_SG_D_3/1
  d_psi_gq_SG_D_3_block/1(Blockout_d_psi_gq_SG_D_3_99f04) -> psi_gq_SG_D_3/1
  Px_3_SG_D_3/1 -> d_V_f_SG_D_3_block/3(State_Px_3_SG_D_3_db85f), d_Px_3_SG_D_3_block/1(State_Px_3_SG_D_3_8e084)
  V_f_SG_D_3/1 -> d_V_f_SG_D_3_block/14(State_V_f_SG_D_3_405ca), d_E_fd_SG_D_3_block/2(State_V_f_SG_D_3_f0dc9)
  d_E_fd_SG_D_3_block/1(Blockout_d_E_fd_SG_D_3_4637c) -> E_fd_SG_D_3/1
  E_fd_SG_D_3/1 -> d_V_f_SG_D_3_block/1(State_E_fd_SG_D_3_2e5ac), d_R_f_SG_D_3_block/1(State_E_fd_SG_D_3_188a8), d_psi_fd_SG_D_3_block/1(State_E_fd_SG_D_3_39d66), d_E_fd_SG_D_3_block/1(State_E_fd_SG_D_3_e3ff2)
  d_psi_fd_SG_D_3_block/1(Blockout_d_psi_fd_SG_D_3_026a9) -> psi_fd_SG_D_3/1

== system case7/AC_1/d_id_line_1_4_block ==
  note: d_id_line_1_4 in case7
      | $376.991118430775\,\mathrm{iq}_{\mathrm{line},1,4}+6520.85548321271\,\mathrm{vd}_{\mathrm{bus},1}-6520.85548321271\,\mathrm{vd}_{\mathrm{bus},4}$
      | Automatically generated on 2025-10-31 19:27:30 .
  State_iq_line_1_4_9d35a : Inport
  State_vd_bus_1_07647 : Inport  Port=2
  State_vd_bus_4_026ae : Inport  Port=3
  Add_15302 : Sum
  Constant_376.991118430775_b734d : Constant  Value=376.991118430775
  Constant_6520.85548321271_0f96c : Constant  Value=6520.85548321271
  Constant_6520.85548321271_2d207 : Constant  Value=6520.85548321271
  Product_0754f : Product
  Product_09995 : Product
  Product_da246 : Product
  Subtract_f1f60 : Sum  Inputs=+-
  Blockout_d_id_line_1_4_c51d9 : Outport
  wires:
  Constant_376.991118430775_b734d/1 -> Product_09995/1
  Product_da246/1 -> Add_15302/2
  State_iq_line_1_4_9d35a/1 -> Product_09995/2
  Subtract_f1f60/1 -> Blockout_d_id_line_1_4_c51d9/1
  Constant_6520.85548321271_2d207/1 -> Product_da246/1
  Product_09995/1 -> Add_15302/1
  State_vd_bus_1_07647/1 -> Product_da246/2
  Constant_6520.85548321271_0f96c/1 -> Product_0754f/1
  State_vd_bus_4_026ae/1 -> Product_0754f/2
  Add_15302/1 -> Subtract_f1f60/1
  Product_0754f/1 -> Subtract_f1f60/2

== system case7/AC_1/d_id_line_3_6_block ==
  note: d_id_line_3_6 in case7
      | $376.991118430775\,\mathrm{iq}_{\mathrm{line},3,6}+6409.57808588826\,\mathrm{vd}_{\mathrm{bus},3}-6409.57808588826\,\mathrm{vd}_{\mathrm{bus},6}$
      | Automatically generated on 2025-10-31 19:27:41 .
  State_iq_line_3_6_444c3 : Inport
  State_vd_bus_3_678dc : Inport  Port=2
  State_vd_bus_6_3dc31 : Inport  Port=3
  Add_46a3a : Sum
  Constant_376.991118430775_868cd : Constant  Value=376.991118430775
  Constant_6409.57808588826_572a8 : Constant  Value=6409.57808588826
  Constant_6409.57808588826_d89fc : Constant  Value=6409.57808588826
  Product_42287 : Product
  Product_5b4e4 : Product
  Product_e2108 : Product
  Subtract_51c84 : Sum  Inputs=+-
  Blockout_d_id_line_3_6_3d598 : Outport
  wires:
  State_vd_bus_3_678dc/1 -> Product_e2108/2
  Constant_376.991118430775_868cd/1 -> Product_42287/1
  Product_e2108/1 -> Add_46a3a/2
  State_iq_line_3_6_444c3/1 -> Product_42287/2
  Constant_6409.57808588826_572a8/1 -> Product_e2108/1
  Product_42287/1 -> Add_46a3a/1
  Constant_6409.57808588826_d89fc/1 -> Product_5b4e4/1
  State_vd_bus_6_3dc31/1 -> Product_5b4e4/2
  Add_46a3a/1 -> Subtract_51c84/1
  Product_5b4e4/1 -> Subtract_51c84/2
  Subtract_51c84/1 -> Blockout_d_id_line_3_6_3d598/1

== system case7/AC_1/d_id_line_4_5_block ==
  note: d_id_line_4_5 in case7
      | $376.991118430775\,\mathrm{iq}_{\mathrm{line},4,5}-68.4144322264777\,\mathrm{id}_{\mathrm{line},4,5}+4082.62256340274\,\mathrm{vd}_{\mathrm{bus},4}-4082.62256340274\,\mathrm{vd}_{\mathrm{bus},5}$
      | Automatically generated on 2025-10-31 19:27:34 .
  State_id_line_4_5_e6f56 : Inport
  State_iq_line_4_5_ed095 : Inport  Port=2
  State_vd_bus_4_76923 : Inport  Port=3
  State_vd_bus_5_748a8 : Inport  Port=4
  Add_00605 : Sum
  Add_c00ca : Sum
  Constant_-68.4144322264777_0e07b : Constant  Value=-68.4144322264777
  Constant_376.991118430775_637f3 : Constant  Value=376.991118430775
  Constant_4082.62256340274_499af : Constant  Value=4082.62256340274
  Constant_4082.62256340274_73445 : Constant  Value=4082.62256340274
  Product_6ef8a : Product
  Product_7b982 : Product
  Product_c9ed3 : Product
  Product_e371f : Product
  Subtract_23144 : Sum  Inputs=+-
  Blockout_d_id_line_4_5_dc71b : Outport
  wires:
  Constant_-68.4144322264777_0e07b/1 -> Product_c9ed3/1
  Product_e371f/1 -> Add_00605/2
  State_id_line_4_5_e6f56/1 -> Product_c9ed3/2
  Constant_376.991118430775_637f3/1 -> Product_e371f/1
  State_iq_line_4_5_ed095/1 -> Product_e371f/2
  Product_c9ed3/1 -> Add_00605/1
  Constant_4082.62256340274_499af/1 -> Product_6ef8a/1
  State_vd_bus_4_76923/1 -> Product_6ef8a/2
  Add_00605/1 -> Add_c00ca/1
  Product_6ef8a/1 -> Add_c00ca/2
  Constant_4082.62256340274_73445/1 -> Product_7b982/1
  State_vd_bus_5_748a8/1 -> Product_7b982/2
  Add_c00ca/1 -> Subtract_23144/1
  Product_7b982/1 -> Subtract_23144/2
  Subtract_23144/1 -> Blockout_d_id_line_4_5_dc71b/1

== system case7/AC_1/d_id_line_5_6_block ==
  note: d_id_line_5_6 in case7
      | $376.991118430775\,\mathrm{iq}_{\mathrm{line},5,6}-84.9380563420768\,\mathrm{id}_{\mathrm{line},5,6}+2209.41926960619\,\mathrm{vd}_{\mathrm{bus},5}-2209.41926960619\,\mathrm{vd}_{\mathrm{bus},6}$
      | Automatically generated on 2025-10-31 19:27:37 .
  State_id_line_5_6_f2138 : Inport
  State_iq_line_5_6_26212 : Inport  Port=2
  State_vd_bus_5_5d5fa : Inport  Port=3
  State_vd_bus_6_92612 : Inport  Port=4
  Add_6a5e2 : Sum
  Add_b3c07 : Sum
  Constant_-84.9380563420768_28db0 : Constant  Value=-84.9380563420768
  Constant_2209.41926960619_21a9a : Constant  Value=2209.41926960619
  Constant_2209.41926960619_faeed : Constant  Value=2209.41926960619
  Constant_376.991118430775_5acb7 : Constant  Value=376.991118430775
  Product_2213b : Product
  Product_2e688 : Product
  Product_4a2df : Product
  Product_ed5c3 : Product
  Subtract_d7560 : Sum  Inputs=+-
  Blockout_d_id_line_5_6_fc4e7 : Outport
  wires:
  Constant_-84.9380563420768_28db0/1 -> Product_ed5c3/1
  Product_4a2df/1 -> Add_6a5e2/2
  State_id_line_5_6_f2138/1 -> Product_ed5c3/2
  Constant_376.991118430775_5acb7/1 -> Product_4a2df/1
  Product_ed5c3/1 -> Add_6a5e2/1
  State_iq_line_5_6_26212/1 -> Product_4a2df/2
  Constant_2209.41926960619_21a9a/1 -> Product_2213b/1
  Product_2e688/1 -> Subtract_d7560/2
  State_vd_bus_5_5d5fa/1 -> Product_2213b/2
  Add_6a5e2/1 -> Add_b3c07/1
  Product_2213b/1 -> Add_b3c07/2
  Constant_2209.41926960619_faeed/1 -> Product_2e688/1
  State_vd_bus_6_92612/1 -> Product_2e688/2
  Add_b3c07/1 -> Subtract_d7560/1
  Subtract_d7560/1 -> Blockout_d_id_line_5_6_fc4e7/1

== system case7/AC_1/d_id_line_6_7_block ==
  note: d_id_line_6_7 in case7
      | $376.991118430775\,\mathrm{iq}_{\mathrm{line},6,7}-43.7092205891385\,\mathrm{id}_{\mathrm{line},6,7}+3726.2031332644\,\mathrm{vd}_{\mathrm{bus},6}-3726.2031332644\,\mathrm{vd}_{\mathrm{bus},7}$
      | Automatically generated on 2025-10-31 19:27:44 .
  State_id_line_6_7_8b489 : Inport
  State_iq_line_6_7_c6725 : Inport  Port=2
  State_vd_bus_6_b4206 : Inport  Port=3
  State_vd_bus_7_b412f : Inport  Port=4
  Add_25cc7 : Sum
  Add_c70d4 : Sum
  Constant_-43.7092205891385_f4695 : Constant  Value=-43.7092205891385
  Constant_3726.2031332644_0b92b : Constant  Value=3726.2031332644
  Constant_3726.2031332644_90c52 : Constant  Value=3726.2031332644
  Constant_376.991118430775_96451 : Constant  Value=376.991118430775
  Product_04fc1 : Product
  Product_29f12 : Product
  Product_2aeb4 : Product
  Product_dfa03 : Product
  Subtract_e1fe6 : Sum  Inputs=+-
  Blockout_d_id_line_6_7_76637 : Outport
  wires:
  Constant_-43.7092205891385_f4695/1 -> Product_dfa03/1
  Product_2aeb4/1 -> Add_c70d4/2
  State_id_line_6_7_8b489/1 -> Product_dfa03/2
  Constant_376.991118430775_96451/1 -> Product_2aeb4/1
  State_iq_line_6_7_c6725/1 -> Product_2aeb4/2
  Product_dfa03/1 -> Add_c70d4/1
  Constant_3726.2031332644_0b92b/1 -> Product_04fc1/1
  State_vd_bus_6_b4206/1 -> Product_04fc1/2
  Add_c70d4/1 -> Add_25cc7/1
  Product_04fc1/1 -> Add_25cc7/2
  Constant_3726.2031332644_90c52/1 -> Product_29f12/1
  State_vd_bus_7_b412f/1 -> Product_29f12/2
  Add_25cc7/1 -> Subtract_e1fe6/1
  Product_29f12/1 -> Subtract_e1fe6/2
  Subtract_e1fe6/1 -> Blockout_d_id_line_6_7_76637/1

== system case7/AC_1/d_id_line_7_8_block ==
  note: d_id_line_7_8 in case7
      | $376.991118430775\,\mathrm{iq}_{\mathrm{line},7,8}-43.7092205891385\,\mathrm{id}_{\mathrm{line},7,8}+5216.68438657017\,\mathrm{vd}_{\mathrm{bus},7}-5216.68438657017\,\mathrm{vd}_{\mathrm{bus},8}$
      | Automatically generated on 2025-10-31 19:27:48 .
  State_id_line_7_8_0f689 : Inport
  State_iq_line_7_8_c6b57 : Inport  Port=2
  State_vd_bus_7_53355 : Inport  Port=3
  State_vd_bus_8_337bf : Inport  Port=4
  Add_90253 : Sum
  Add_ed008 : Sum
  Constant_-43.7092205891385_b6ebe : Constant  Value=-43.7092205891385
  Constant_376.991118430775_a864b : Constant  Value=376.991118430775
  Constant_5216.68438657017_970b6 : Constant  Value=5216.68438657017
  Constant_5216.68438657017_fee05 : Constant  Value=5216.68438657017
  Product_51fd8 : Product
  Product_955f7 : Product
  Product_cace0 : Product
  Product_f2216 : Product
  Subtract_bd886 : Sum  Inputs=+-
  Blockout_d_id_line_7_8_0c425 : Outport
  wires:
  Constant_-43.7092205891385_b6ebe/1 -> Product_f2216/1
  Product_51fd8/1 -> Add_90253/2
  State_id_line_7_8_0f689/1 -> Product_f2216/2
  Constant_376.991118430775_a864b/1 -> Product_51fd8/1
  Product_f2216/1 -> Add_90253/1
  State_iq_line_7_8_c6b57/1 -> Product_51fd8/2
  Constant_5216.68438657017_fee05/1 -> Product_cace0/1
  State_vd_bus_7_53355/1 -> Product_cace0/2
  Add_90253/1 -> Add_ed008/1
  Product_cace0/1 -> Add_ed008/2
  Constant_5216.68438657017_970b6/1 -> Product_955f7/1
  State_vd_bus_8_337bf/1 -> Product_955f7/2
  Add_ed008/1 -> Subtract_bd886/1
  Product_955f7/1 -> Subtract_bd886/2
  Subtract_bd886/1 -> Blockout_d_id_line_7_8_0c425/1

== system case7/AC_1/d_id_line_8_2_block ==
  note: d_id_line_8_2 in case7
      | $376.991118430775\,\mathrm{iq}_{\mathrm{line},8,2}-6009.62041332883\,\mathrm{vd}_{\mathrm{bus},2}+6009.62041332883\,\mathrm{vd}_{\mathrm{bus},8}$
      | Automatically generated on 2025-10-31 19:27:52 .
  State_iq_line_8_2_8eb85 : Inport
  State_vd_bus_2_e858e : Inport  Port=2
  State_vd_bus_8_0adbc : Inport  Port=3
  Add_4041a : Sum
  Constant_376.991118430775_0f759 : Constant  Value=376.991118430775
  Constant_6009.62041332883_8e806 : Constant  Value=6009.62041332883
  Constant_6009.62041332883_b13b6 : Constant  Value=6009.62041332883
  Product_08563 : Product
  Product_0cf2b : Product
  Product_f5cbe : Product
  Subtract_f7bdc : Sum  Inputs=+-
  Blockout_d_id_line_8_2_4b586 : Outport
  wires:
  State_vd_bus_2_e858e/1 -> Product_0cf2b/2
  Constant_376.991118430775_0f759/1 -> Product_08563/1
  Product_0cf2b/1 -> Subtract_f7bdc/2
  State_iq_line_8_2_8eb85/1 -> Product_08563/2
  Constant_6009.62041332883_8e806/1 -> Product_0cf2b/1
  Product_08563/1 -> Subtract_f7bdc/1
  Constant_6009.62041332883_b13b6/1 -> Product_f5cbe/1
  State_vd_bus_8_0adbc/1 -> Product_f5cbe/2
  Subtract_f7bdc/1 -> Add_4041a/1
  Product_f5cbe/1 -> Add_4041a/2
  Add_4041a/1 -> Blockout_d_id_line_8_2_4b586/1

== system case7/AC_1/d_id_line_8_9_block ==
  note: d_id_line_8_9 in case7
      | $376.991118430775\,\mathrm{iq}_{\mathrm{line},8,9}-73.5886329831021\,\mathrm{id}_{\mathrm{line},8,9}+2332.92717908728\,\mathrm{vd}_{\mathrm{bus},8}-2332.92717908728\,\mathrm{vd}_{\mathrm{bus},9}$
      | Automatically generated on 2025-10-31 19:27:55 .
  State_id_line_8_9_6c653 : Inport
  State_iq_line_8_9_a7084 : Inport  Port=2
  State_vd_bus_8_dd79d : Inport  Port=3
  State_vd_bus_9_2283c : Inport  Port=4
  Add_5d950 : Sum
  Add_a2a56 : Sum
  Constant_-73.5886329831021_13659 : Constant  Value=-73.5886329831021
  Constant_2332.92717908728_5c247 : Constant  Value=2332.92717908728
  Constant_2332.92717908728_f5ead : Constant  Value=2332.92717908728
  Constant_376.991118430775_a8ccd : Constant  Value=376.991118430775
  Product_1b3f5 : Product
  Product_510d5 : Product
  Product_aea9b : Product
  Product_f9599 : Product
  Subtract_93cab : Sum  Inputs=+-
  Blockout_d_id_line_8_9_f11ed : Outport
  wires:
  Constant_-73.5886329831021_13659/1 -> Product_1b3f5/1
  Product_aea9b/1 -> Add_5d950/2
  State_id_line_8_9_6c653/1 -> Product_1b3f5/2
  Constant_376.991118430775_a8ccd/1 -> Product_aea9b/1
  State_iq_line_8_9_a7084/1 -> Product_aea9b/2
  Product_1b3f5/1 -> Add_5d950/1
  Constant_2332.92717908728_f5ead/1 -> Product_f9599/1
  State_vd_bus_8_dd79d/1 -> Product_f9599/2
  Add_5d950/1 -> Add_a2a56/1
  Product_f9599/1 -> Add_a2a56/2
  Constant_2332.92717908728_5c247/1 -> Product_510d5/1
  State_vd_bus_9_2283c/1 -> Product_510d5/2
  Add_a2a56/1 -> Subtract_93cab/1
  Product_510d5/1 -> Subtract_93cab/2
  Subtract_93cab/1 -> Blockout_d_id_line_8_9_f11ed/1

== system case7/AC_1/d_id_line_9_4_block ==
  note: d_id_line_9_4 in case7
      | $376.991118430775\,\mathrm{iq}_{\mathrm{line},9,4}-43.5579776113214\,\mathrm{id}_{\mathrm{line},9,4}-4418.83853921238\,\mathrm{vd}_{\mathrm{bus},4}+4418.83853921238\,\mathrm{vd}_{\mathrm{bus},9}$
      | Automatically generated on 2025-10-31 19:27:59 .
  State_id_line_9_4_e74bb : Inport
  State_iq_line_9_4_d6adc : Inport  Port=2
  State_vd_bus_4_536cf : Inport  Port=3
  State_vd_bus_9_20c24 : Inport  Port=4
  Add_404e9 : Sum
  Add_8a3f2 : Sum
  Constant_-43.5579776113214_a7c48 : Constant  Value=-43.5579776113214
  Constant_376.991118430775_9a522 : Constant  Value=376.991118430775
  Constant_4418.83853921238_3a2f6 : Constant  Value=4418.83853921238
  Constant_4418.83853921238_7b9d8 : Constant  Value=4418.83853921238
  Product_149be : Product
  Product_18769 : Product
  Product_47ea6 : Product
  Product_7aece : Product
  Subtract_4501b : Sum  Inputs=+-
  Blockout_d_id_line_9_4_76f50 : Outport
  wires:
  Constant_-43.5579776113214_a7c48/1 -> Product_149be/1
  Product_18769/1 -> Add_8a3f2/2
  State_id_line_9_4_e74bb/1 -> Product_149be/2
  Constant_376.991118430775_9a522/1 -> Product_18769/1
  Product_149be/1 -> Add_8a3f2/1
  State_iq_line_9_4_d6adc/1 -> Product_18769/2
  Constant_4418.83853921238_7b9d8/1 -> Product_47ea6/1
  State_vd_bus_4_536cf/1 -> Product_47ea6/2
  Add_8a3f2/1 -> Subtract_4501b/1
  Product_47ea6/1 -> Subtract_4501b/2
  Constant_4418.83853921238_3a2f6/1 -> Product_7aece/1
  Subtract_4501b/1 -> Add_404e9/1
  State_vd_bus_9_20c24/1 -> Product_7aece/2
  Product_7aece/1 -> Add_404e9/2
  Add_404e9/1 -> Blockout_d_id_line_9_4_76f50/1

== system case7/AC_1/d_id_load_5_block ==
  note: d_id_load_5 in case7
      | $376.991118430775\,\mathrm{iq}_{\mathrm{load},5}-1242.47744681877\,\mathrm{id}_{\mathrm{load},5}+1265.54551301855\,\mathrm{vd}_{\mathrm{bus},5}$
      | Automatically generated on 2025-10-31 19:27:20 .
  State_id_load_5_77b25 : Inport
  State_iq_load_5_98165 : Inport  Port=2
  State_vd_bus_5_6eea2 : Inport  Port=3
  Add_1325b : Sum
  Add_bed07 : Sum
  Constant_-1242.47744681877_3d19d : Constant  Value=-1242.47744681877
  Constant_1265.54551301855_9b4b0 : Constant  Value=1265.54551301855
  Constant_376.991118430775_71616 : Constant  Value=376.991118430775
  Product_6d994 : Product
  Product_747ef : Product
  Product_d6191 : Product
  Blockout_d_id_load_5_06c96 : Outport
  wires:
  Constant_-1242.47744681877_3d19d/1 -> Product_6d994/1
  Product_747ef/1 -> Add_bed07/2
  State_id_load_5_77b25/1 -> Product_6d994/2
  Constant_376.991118430775_71616/1 -> Product_747ef/1
  Product_d6191/1 -> Add_1325b/2
  State_iq_load_5_98165/1 -> Product_747ef/2
  Product_6d994/1 -> Add_bed07/1
  Constant_1265.54551301855_9b4b0/1 -> Product_d6191/1
  State_vd_bus_5_6eea2/1 -> Product_d6191/2
  Add_bed07/1 -> Add_1325b/1
  Add_1325b/1 -> Blockout_d_id_load_5_06c96/1
